simulink model "Commande_Vitesse_v2"  (R2024b)
settings: Solver=VariableStepAuto  StartTime=0.0  StopTime=.6  RelTol=1e-3
undefined symbols (not defined in the file): g, Isat, Jeq, Kc, Kii_EPOS, Kip_EPOS, KIv_EPOS, KPv_EPOS, kr, Lm, Mtot, r, rkr, Rm, Usat
settings Model: Creator=xpess  LastModifiedBy=xpess
settings SolverCC: ZeroCrossAlgorithm=Adaptive
settings DebuggingCC: IgnoredZcDiagnostic=none
settings RTWCC: GPUComputeCapability=3.5

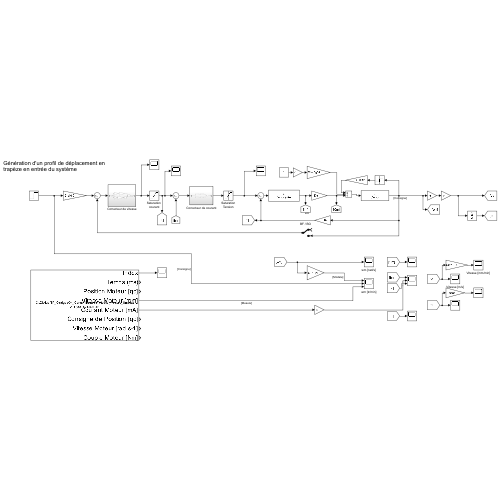
[thumbnail: Simulink's stored preview of the top-level diagram]
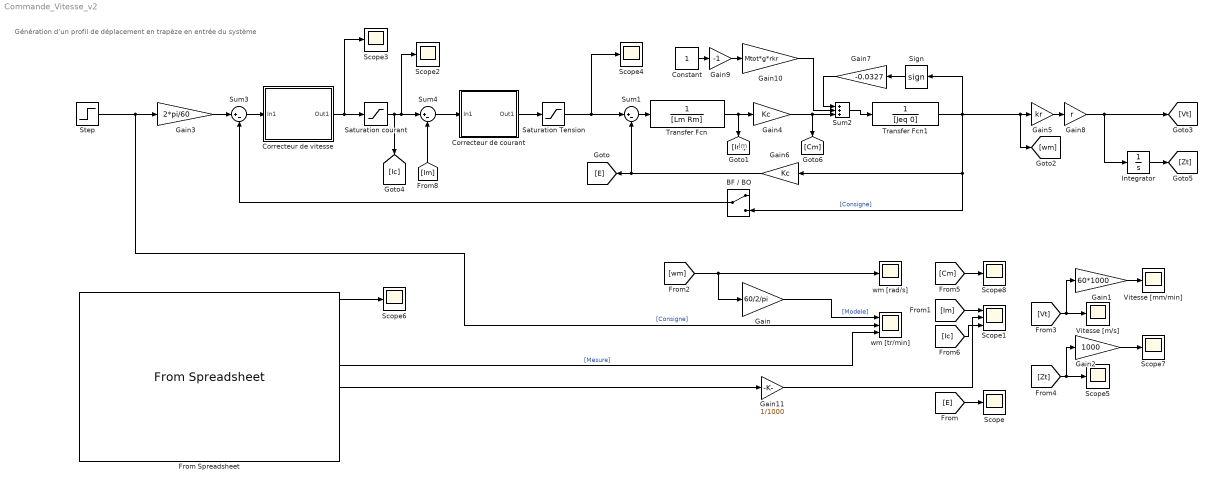
== system Commande_Vitesse_v2 ==
  note: Im
  note: Génération d'un profil de déplacement en trapèze en entrée du système
  BF / BO : ManualSwitch
  Constant : Constant
  Correcteur de courant : Subsystem
  Correcteur de vitesse : Subsystem
  From Spreadsheet : FromSpreadsheet  FileName=C:\GitHub\TP_Corriges\04_Comax\Mesures\Vitesse_Montee_0m.xlsx  SheetName=V_4000_0mMATLAB  Range=A1:I74
  Gain : Gain  Gain=60/2/pi
  Gain1 : Gain  Gain=60*1000
  Gain10 : Gain  Gain=Mtot*g*rkr
  Gain11 : Gain  Gain=1/1000
  Gain2 : Gain  Gain=1000
  Gain3 : Gain  Gain=2*pi/60
  Gain4 : Gain  Gain=Kc
  Gain5 : Gain  Gain=kr
  Gain6 : Gain  Gain=Kc
  Gain7 : Gain  Gain=-0.0327
  Gain8 : Gain  Gain=r
  Gain9 : Gain  Gain=-1
  Integrator : Integrator
  Saturation Tension : Saturate  UpperLimit=Usat  LowerLimit=-Usat
  Saturation courant : Saturate  UpperLimit=Isat  LowerLimit=-Isat
  Scope{,2..8} (8 alike) : Scope
  Scope1 : Scope  NumInputPorts=3
  Sign : Signum
  Step : Step  Time=.137*0  After=4000  SampleTime=0
  Sum1 : Sum  Inputs=|+-
  Sum2 : Sum  Inputs=+++
  Sum3 : Sum  Inputs=|+-
  Sum4 : Sum  Inputs=|+-
  Transfer Fcn : TransferFcn  Denominator=[Lm Rm]
  Transfer Fcn1 : TransferFcn  Denominator=[Jeq 0]
  Vitesse [m/s] : Scope
  Vitesse [mm/min] : Scope
  wm [rad/s] : Scope
  wm [tr/min] : Scope  NumInputPorts=3
  wires:
  Gain6/1 -> Sum1/2, [E]
  [E] -> Scope/1
  [Im] -> Scope1/1
  [wm] -> Gain/1, wm [rad/s]/1
  Gain/1 -> wm [tr/min]/1  "[Modele]"
  [Vt] -> Gain1/1, Vitesse [m/s]/1
  [Zt] -> Gain2/1, Scope5/1
  Gain1/1 -> Vitesse [mm/min]/1
  Gain2/1 -> Scope7/1
  [Cm] -> Scope8/1
  Step/1 -> Gain3/1, wm [tr/min]/2  "[Consigne]"
  Gain3/1 -> Sum3/1
  BF / BO/1 -> Sum3/2
  [Im] -> Sum4/2
  Sum4/1 -> Correcteur de courant/1(In1)
  From Spreadsheet/1 -> Scope6/1
  From Spreadsheet/4 -> wm [tr/min]/3  "[Mesure]"
  Saturation courant/1 -> [Ic], Sum4/1, Scope2/1
  Transfer Fcn/1 -> [Im], Gain4/1
  Gain4/1 -> [Cm], Sum2/3
  Sum1/1 -> Transfer Fcn/1
  Gain5/1 -> Gain8/1
  Gain8/1 -> [Vt], Integrator/1
  Integrator/1 -> [Zt]
  Sum2/1 -> Transfer Fcn1/1
  Gain10/1 -> Sum2/2
  Gain9/1 -> Gain10/1
  Transfer Fcn1/1 -> Gain6/1, BF / BO/2, Sign/1, Gain5/1, [wm]  "[Consigne]"
  Constant/1 -> Gain9/1
  Correcteur de courant/1(Out1) -> Saturation Tension/1
  Sign/1 -> Gain7/1
  Gain7/1 -> Sum2/1
  Saturation Tension/1 -> Scope4/1, Sum1/1
  From Spreadsheet/5 -> Gain11/1
  Gain11/1 -> Scope1/2
  [Ic] -> Scope1/3
  Sum3/1 -> Correcteur de vitesse/1(In1)
  Correcteur de vitesse/1(Out1) -> Scope3/1, Saturation courant/1

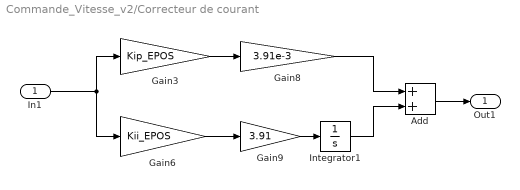
== system Commande_Vitesse_v2/Correcteur de courant ==
  In1 : Inport
  Add : Sum
  Gain3 : Gain  Gain=Kip_EPOS
  Gain6 : Gain  Gain=Kii_EPOS
  Gain8 : Gain  Gain=3.91e-3
  Gain9 : Gain  Gain=3.91
  Integrator1 : Integrator
  Out1 : Outport
  wires:
  Gain9/1 -> Integrator1/1
  In1/1 -> Gain6/1, Gain3/1
  Add/1 -> Out1/1
  Integrator1/1 -> Add/2
  Gain6/1 -> Gain9/1
  Gain8/1 -> Add/1
  Gain3/1 -> Gain8/1

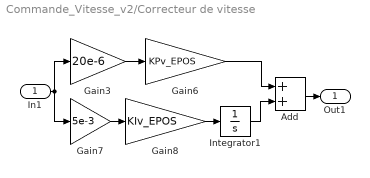
== system Commande_Vitesse_v2/Correcteur de vitesse ==
  In1 : Inport
  Add : Sum
  Gain3 : Gain  Gain=20e-6
  Gain6 : Gain  Gain=KPv_EPOS
  Gain7 : Gain  Gain=5e-3
  Gain8 : Gain  Gain=KIv_EPOS
  Integrator1 : Integrator
  Out1 : Outport
  wires:
  Gain8/1 -> Integrator1/1
  Add/1 -> Out1/1
  Gain3/1 -> Gain6/1
  Integrator1/1 -> Add/2
  In1/1 -> Gain7/1, Gain3/1
  Gain6/1 -> Add/1
  Gain7/1 -> Gain8/1
